simulink model "ysw15_1"  (R2014a)
settings: Solver=ode45  StartTime=0.0  StopTime=10.0  RelTol=1e-3
undefined symbols (not defined in the file or in its folder): hylv
settings Model: Creator=ii  LastModifiedBy=ii
settings SolverCC: ZeroCrossAlgorithm=Adaptive
settings DebuggingCC: UnderspecifiedInitializationDetection=Classic

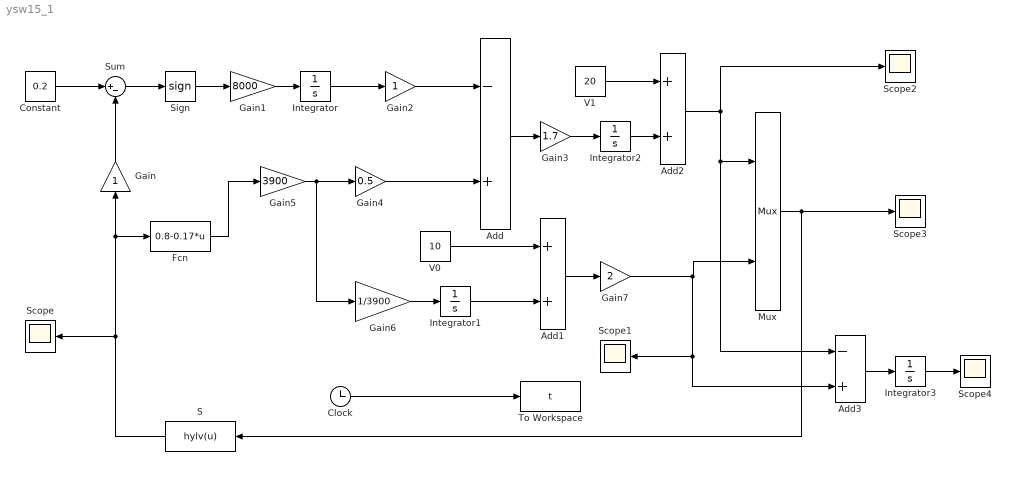
== system ysw15_1 ==
  Add : Sum  Inputs=-+
  Add1 : Sum
  Add2 : Sum
  Add3 : Sum  Inputs=-+
  Clock : Clock
  Constant : Constant  Value=0.2
  Fcn : Fcn  Expr=0.8-0.17*u
  Gain : Gain
  Gain1 : Gain  Gain=8000
  Gain2 : Gain
  Gain3 : Gain  Gain=1.7
  Gain4 : Gain  Gain=0.5
  Gain5 : Gain  Gain=3900
  Gain6 : Gain  Gain=1/3900
  Gain7 : Gain  Gain=2
  Integrator{,1..3} (4 alike) : Integrator
  Mux : Mux  Inputs=2
  S : MATLABFcn  MATLABFcn=hylv(u)
  Scope{,1..4} (5 alike) : Scope
      Scope2 settings: SaveName=ScopeData2
      Scope3 settings: SaveName=ScopeData3
      Scope4 settings: SaveName=ScopeData4
  Sign : Signum
  Sum : Sum  Inputs=|+-
  To Workspace : ToWorkspace  VariableName=t  SampleTime=-1
  V0 : Constant  Value=10
  V1 : Constant  Value=20
  wires:
  Constant/1 -> Sum/1
  Gain/1 -> Sum/2
  Sum/1 -> Sign/1
  Sign/1 -> Gain1/1
  Gain1/1 -> Integrator/1
  Integrator/1 -> Gain2/1
  Gain2/1 -> Add/1
  Add/1 -> Gain3/1
  Gain4/1 -> Add/2
  Gain5/1 -> Gain6/1, Gain4/1
  Fcn/1 -> Gain5/1
  Clock/1 -> To Workspace/1
  Gain6/1 -> Integrator1/1
  V0/1 -> Add1/1
  Integrator1/1 -> Add1/2
  Gain3/1 -> Integrator2/1
  V1/1 -> Add2/1
  Integrator2/1 -> Add2/2
  Add1/1 -> Gain7/1
  S/1 -> Fcn/1, Gain/1, Scope/1
  Add2/1 -> Add3/1, Mux/1, Scope2/1
  Gain7/1 -> Mux/2, Add3/2, Scope1/1
  Mux/1 -> S/1, Scope3/1
  Add3/1 -> Integrator3/1
  Integrator3/1 -> Scope4/1
